simulink model "linear_fil"  (R2020a)
settings: Solver=VariableStepAuto  StartTime=0.0  StopTime=10.0  RelTol=1e-3
settings Model: Creator=Shubham  LastModifiedBy=Shubham

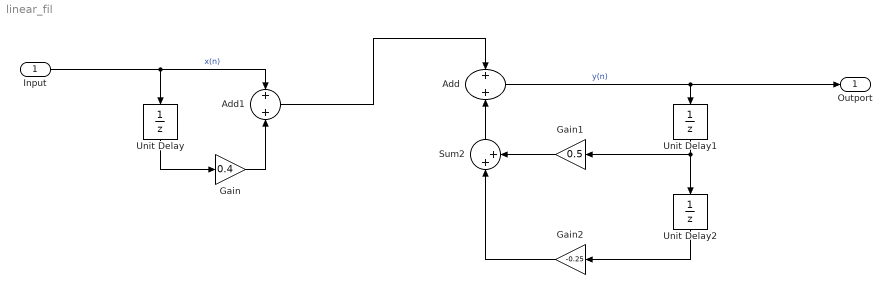
== system linear_fil ==
  Input : Inport
  Add : Sum
  Add1 : Sum
  Gain : Gain  Gain=0.4
  Gain1 : Gain  Gain=0.5
  Gain2 : Gain  Gain=-0.25
  Sum2 : Sum  Inputs=|++
  Unit Delay : UnitDelay  SampleTime=-1  HasFrameUpgradeWarning=on
  Unit Delay1 : UnitDelay  SampleTime=-1  HasFrameUpgradeWarning=on
  Unit Delay2 : UnitDelay  SampleTime=-1  HasFrameUpgradeWarning=on
  Outport : Outport
  wires:
  Unit Delay/1 -> Gain/1
  Sum2/1 -> Add/2
  Gain1/1 -> Sum2/2
  Unit Delay2/1 -> Gain2/1
  Gain2/1 -> Sum2/1
  Input/1 -> Add1/1, Unit Delay/1  "x(n)"
  Gain/1 -> Add1/2
  Add1/1 -> Add/1
  Add/1 -> Unit Delay1/1, Outport/1  "y(n)"
  Unit Delay1/1 -> Unit Delay2/1, Gain1/1
